simulink model "UPI_CC_3ph_4w_seq_23b"  (R2023b)
settings: Solver=FixedStepDiscrete  StartTime=0.0  StopTime=15  FixedStep=Ts_Power  MaxStep=1e-4  RelTol=1e-3
InitFcn:
  | run PI_OL_vs_UPI_CC_sec_ini;
undefined symbols (not defined in the file): C_2, DiscIntNeverNeededParam, K_i_pll, K_iv, K_p_pll, Ki_i, Kp_i, Kp_v, L_n, L_s2, L_t, L_t2, params_cc, params_pi_cc, params_pi_vc, params_vc_cc, R_d2, R_n, R_s2, R_t2, S_b, Ts_Control, Ts_Power, v_dc
libraries: spsFirstOrderFilterLib x7, spsThreePhaseSeriesRLCBranchLib x5, spsSeriesRLCLoadLib x5, spsUniversalBridgeLib x5, spsControlledVoltageSourceLib x3, spsThreePhaseVIMeasurementLib x3, eeGeneralControl x2, spsPower3phInstantaneousLib x2, spsSeriesRLCBranchLib x2, spsThreePhaseBreakerLib x2, spsRMSLib x1, simulink x1
(part 1 of 2)
settings Model: Creator=Manuel  LastModifiedBy=manba
settings SolverCC: AlgebraicLoopSolver=TrustRegion
settings DataIOCC: ReturnWorkspaceOutputs=off
settings DebuggingCC: UnconnectedInputMsg=warning  UnconnectedOutputMsg=warning  UnconnectedLineMsg=warning  ArithmeticOperatorsInVariantConditions=warning
settings ModelReferenceCC: EnableRefExpFcnMdlSchedulingChecks=on
settings SFSimCC: SimUseLocalCustomCode=off  CustomCodeUndefinedFunction=UseInterfaceOnly
settings RTWCC: RTWUseLocalCustomCode=off  DLArmComputeVersion=19.05

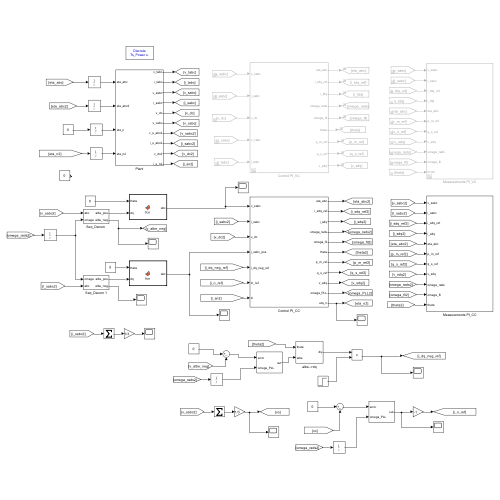
[thumbnail: Simulink's stored preview of the top-level diagram]
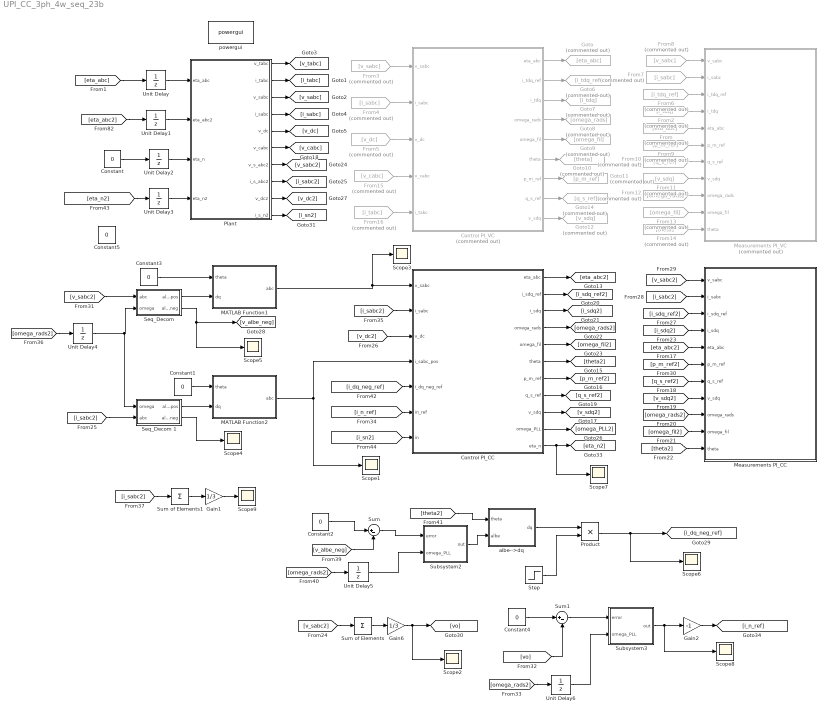
== system UPI_CC_3ph_4w_seq_23b ==
  Constant{,1..5} (6 alike) : Constant  Value=0
  Control PI_CC : Subsystem
  Control PI_VC : Subsystem  Commented=on
  From : From  Commented=on  GotoTag=eta_abc
  From10 : From  Commented=on  GotoTag=q_s_ref
  From11 : From  Commented=on  GotoTag=v_sdq
  From12 : From  Commented=on  GotoTag=omega_rads
  From13 : From  Commented=on  GotoTag=omega_fil
  From14 : From  Commented=on  GotoTag=theta
  From15 : From  Commented=on  GotoTag=v_cabc
  From16 : From  Commented=on  GotoTag=i_tabc
  From2 : From  Commented=on  GotoTag=i_tdq
  From3 : From  Commented=on  GotoTag=v_sabc
  From4 : From  Commented=on  GotoTag=i_sabc
  From5 : From  Commented=on  GotoTag=v_dc
  From6 : From  Commented=on  GotoTag=i_tdq_ref
  From7 : From  Commented=on  GotoTag=i_sabc
  From8 : From  Commented=on  GotoTag=v_sabc
  From9 : From  Commented=on  GotoTag=p_m_ref
  Gain1 : Gain  Gain=1/3
  Gain2 : Gain  Gain=-1
  Gain6 : Gain  Gain=1/3
  Goto : Goto  Commented=on  GotoTag=eta_abc
  Goto10 : Goto  Commented=on  GotoTag=theta
  Goto11 : Goto  Commented=on  GotoTag=p_m_ref
  Goto12 : Goto  Commented=on  GotoTag=v_sdq
  Goto14 : Goto  Commented=on  GotoTag=q_s_ref
  Goto6 : Goto  Commented=on  GotoTag=i_tdq_ref
  Goto7 : Goto  Commented=on  GotoTag=i_tdq
  Goto8 : Goto  Commented=on  GotoTag=omega_rads
  Goto9 : Goto  Commented=on  GotoTag=omega_fil
  MATLAB Function1 : MATLAB Function  TreatAsAtomicUnit=on
  MATLAB Function2 : MATLAB Function  TreatAsAtomicUnit=on
  Measurements PI_CC : Subsystem
  Measurements PI_VC : Subsystem  Commented=on
  Plant : Subsystem
  Product : Product
  Scope{1..9} (9 alike) : Scope
  "Seq_Decom " : Subsystem
  Seq_Decom 1 : Subsystem
  Step : Step  Time=7  SampleTime=0
  Subsystem2 : Subsystem
  Subsystem3 : Subsystem
  Sum : Sum  Inputs=|+-
  Sum of Elements : Sum  Inputs=+
  Sum of Elements1 : Sum  Inputs=+
  Sum1 : Sum  Inputs=|+-
  Unit Delay{,1..6} (7 alike) : UnitDelay  SampleTime=-1  HasFrameUpgradeWarning=on
  albe-->dq : Subsystem
  powergui : spspowerguiLib/powergui  Priority=1  SimulationMode=Discrete  SampleTime=Ts_Power  frequency=60  Iterations=50  frequencyindice=0  Pbase=100e6  ErrMax=1e-4  UnitsV=kV  UnitsW=MW  buscounter=0  FunctionMessages=off  echomessages=off  EnableUseOfTLC=off  CurrentSourceSwitches=off  DisableSnubberDevices=off  DisableRonSwitches=off  DisableVfSwitches=off  DisplayEquations=off  AutomaticDiscreteSolvers=off  SolverType=Tustin/Backward Euler (TBE)  Interpol=off  ExternalGateDelay=off  methode=off  Ts=100  x0status=blocks  SPID=on  SwTol=0  HookPort=off  NonlinearTolerance=1e-4  nMaxIteration=100  ContinueOnMaxIteration=off  RestoreLinks=warning  ResistiveCurrentMeasurement=off  Frange=[0:2:500]  Ylog=off  Xlog=on  ShowGrid=off  save=off  variable=ZData  structure=v_sabc  ZoomFFT=off  StartTime=4  cycles=5  DisplayStyle=2  fundamental=50  FreqAxis=off  MaxFrequency=10000  frequencyindicesteady=1  RmsSteady=1  display=off
  wires:
  From3/1 -> Control PI_VC/1(v_sabc)
  From4/1 -> Control PI_VC/2(i_sabc)
  From5/1 -> Control PI_VC/3(v_dc)
  Control PI_VC/1(eta_abc) -> Goto/1
  Control PI_VC/2(i_tdq_ref) -> Goto6/1
  Control PI_VC/3(i_tdq) -> Goto7/1
  Control PI_VC/4(omega_rads) -> Goto8/1
  Control PI_VC/5(omega_fil) -> Goto9/1
  Control PI_VC/6(theta) -> Goto10/1
  Control PI_VC/7(p_m_ref) -> Goto11/1
  Control PI_VC/8(q_s_ref) -> Goto14/1
  Control PI_VC/9(v_sdq) -> Goto12/1
  From/1 -> Measurements PI_VC/5(eta_abc)
  From2/1 -> Measurements PI_VC/4(i_tdq)
  From6/1 -> Measurements PI_VC/3(i_tdq_ref)
  From7/1 -> Measurements PI_VC/2(i_sabc)
  From8/1 -> Measurements PI_VC/1(v_sabc)
  From9/1 -> Measurements PI_VC/6(p_m_ref)
  From10/1 -> Measurements PI_VC/7(q_s_ref)
  From11/1 -> Measurements PI_VC/8(v_sdq)
  From12/1 -> Measurements PI_VC/9(omega_rads)
  From13/1 -> Measurements PI_VC/10(omega_fil)
  From14/1 -> Measurements PI_VC/11(theta)
  From15/1 -> Control PI_VC/4(v_cabc)
  From16/1 -> Control PI_VC/5(i_tabc)
  Plant/2(i_tabc) -> [i_tabc]
  Plant/6(v_cabc) -> [v_cabc]
  [eta_abc] -> Unit Delay/1
  Plant/7(v_s_abc2) -> [v_sabc2]
  Plant/9(v_dc2) -> [v_dc2]
  Constant/1 -> Unit Delay2/1
  Unit Delay/1 -> Plant/1(eta_abc)
  Plant/5(v_dc) -> [v_dc]
  Unit Delay1/1 -> Plant/2(eta_abc2)
  Plant/8(i_s_abc2) -> [i_sabc2]
  Plant/3(v_sabc) -> [v_sabc]
  Plant/1(v_tabc) -> [v_tabc]
  Plant/4(i_sabc) -> [i_sabc]
  Unit Delay2/1 -> Plant/3(eta_n)
  Unit Delay3/1 -> Plant/4(eta_n2)
  [eta_abc2] -> Unit Delay1/1
  Unit Delay5/1 -> Subsystem2/2(omega_PLL)
  Sum/1 -> Subsystem2/1(error)
  "Seq_Decom "/2(albe_neg) -> Scope5/1, [v_albe_neg]
  [i_dq_neg_ref] -> Control PI_CC/5(i_dq_neg_ref)
  [omega_rads2] -> Unit Delay5/1
  [v_albe_neg] -> Sum/2
  [omega_rads2] -> Measurements PI_CC/9(omega_rads)
  MATLAB Function1/1(abc) -> Control PI_CC/1(v_sabc), Scope3/1
  MATLAB Function2/1(abc) -> Scope1/1, Control PI_CC/4(i_sabc_pos)
  "Seq_Decom "/1(albe_pos) -> MATLAB Function1/2(dq)
  Control PI_CC/2(i_sdq_ref) -> [i_sdq_ref2]
  [i_sabc2] -> Seq_Decom 1/2(abc)
  Seq_Decom 1/2(albe_neg) -> Scope4/1
  [v_dc2] -> Control PI_CC/3(v_dc)
  [i_sabc2] -> Measurements PI_CC/2(i_sabc)
  Constant3/1 -> MATLAB Function1/1(theta)
  [v_sabc2] -> "Seq_Decom "/1(abc)
  [i_sabc2] -> Control PI_CC/2(i_sabc)
  [p_m_ref2] -> Measurements PI_CC/6(p_m_ref)
  [q_s_ref2] -> Measurements PI_CC/7(q_s_ref)
  [v_sdq2] -> Measurements PI_CC/8(v_sdq)
  [theta2] -> albe-->dq/1(theta)
  [i_sdq2] -> Measurements PI_CC/4(i_sdq)
  Unit Delay4/1 -> "Seq_Decom "/2(omega), Seq_Decom 1/1(omega)
  [omega_fil2] -> Measurements PI_CC/10(omega_fil)
  [eta_abc2] -> Measurements PI_CC/5(eta_abc)
  Control PI_CC/6(theta) -> [theta2]
  [omega_rads2] -> Unit Delay4/1
  Constant1/1 -> MATLAB Function2/1(theta)
  Control PI_CC/4(omega_rads) -> [omega_rads2]
  Control PI_CC/10(omega_PLL) -> [omega_PLL2]
  Control PI_CC/1(eta_abc) -> [eta_abc2]
  Seq_Decom 1/1(albe_pos) -> MATLAB Function2/2(dq)
  Control PI_CC/3(i_sdq) -> [i_sdq2]
  [theta2] -> Measurements PI_CC/11(theta)
  Control PI_CC/5(omega_fil) -> [omega_fil2]
  [i_sdq_ref2] -> Measurements PI_CC/3(i_sdq_ref)
  Control PI_CC/8(q_s_ref) -> [q_s_ref2]
  Constant2/1 -> Sum/1
  Control PI_CC/9(v_sdq) -> [v_sdq2]
  Subsystem2/1(out) -> albe-->dq/2(albe)
  [v_sabc2] -> Measurements PI_CC/1(v_sabc)
  Control PI_CC/7(p_m_ref) -> [p_m_ref2]
  Sum of Elements/1 -> Gain6/1
  Gain6/1 -> Scope2/1, [vo]
  [v_sabc2] -> Sum of Elements/1
  Constant4/1 -> Sum1/1
  [vo] -> Sum1/2
  Sum1/1 -> Subsystem3/1(error)
  [omega_rads2] -> Unit Delay6/1
  Unit Delay6/1 -> Subsystem3/2(omega_PLL)
  Subsystem3/1(out) -> Scope8/1, Gain2/1
  Plant/10(i_s_n2) -> [i_sn2]
  [i_n_ref] -> Control PI_CC/6(in_ref)
  [i_sn2] -> Control PI_CC/7(in)
  Control PI_CC/11(eta_n) -> Scope7/1, [eta_n2]
  [eta_n2] -> Unit Delay3/1
  [i_sabc2] -> Sum of Elements1/1
  Sum of Elements1/1 -> Gain1/1
  Gain1/1 -> Scope9/1
  Gain2/1 -> [i_n_ref]
  Step/1 -> Product/2
  albe-->dq/1(dq) -> Product/1
  Product/1 -> Scope6/1, [i_dq_neg_ref]

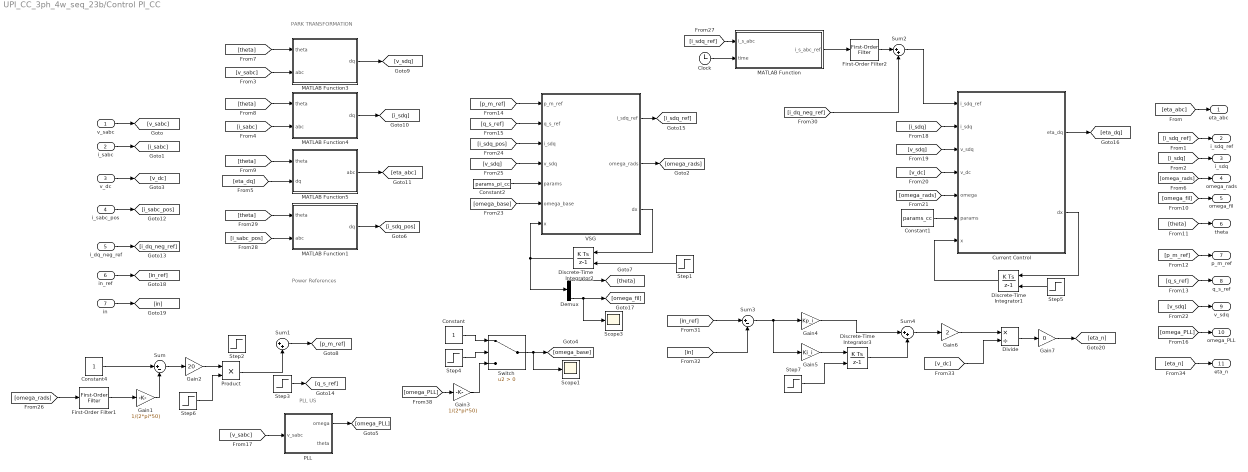
== system UPI_CC_3ph_4w_seq_23b/Control PI_CC ==
  note: PARK TRANSFORMATION
  note: Power References
  note: PLL US
  v_sabc : Inport
  i_sabc : Inport  Port=2
  v_dc : Inport  Port=3
  i_sabc_pos : Inport  Port=4
  i_dq_neg_ref : Inport  Port=5
  in_ref : Inport  Port=6
  in : Inport  Port=7
  Clock : Clock
  Constant : Constant
  Constant1 : Constant  Value=params_cc
  Constant2 : Constant  Value=params_pi_cc
  Constant4 : Constant
  Current Control : MATLAB Function  TreatAsAtomicUnit=on
  Demux : Demux
  Discrete-Time Integrator1 : DiscreteIntegrator  ExternalReset=rising  InitialCondition=[0;0]  SampleTime=Ts_Control  ICPrevOutput=DiscIntNeverNeededParam  ICPrevScaledInput=DiscIntNeverNeededParam
  Discrete-Time Integrator2 : DiscreteIntegrator  ExternalReset=rising  InitialCondition=[0;0;0;2*pi*50]  SampleTime=Ts_Control  ICPrevOutput=DiscIntNeverNeededParam  ICPrevScaledInput=DiscIntNeverNeededParam
  Discrete-Time Integrator3 : DiscreteIntegrator  ExternalReset=rising  SampleTime=Ts_Control  ICPrevOutput=DiscIntNeverNeededParam  ICPrevScaledInput=DiscIntNeverNeededParam
  Divide : Product  Inputs=*/
  First-Order Filter1 : spsFirstOrderFilterLib/First-Order Filter  FilterType=Lowpass  Tc=10e-3  Ts=Ts_Control  Initialize=on  Vac_Init=[0, 0, 60]  Vdc_Init=0  PlotResponse=off  FreqRange="[0,  200,  1]"
  First-Order Filter2 : spsFirstOrderFilterLib/First-Order Filter  FilterType=Lowpass  Tc=2.4e-3  Ts=Ts_Control  Initialize=on  Vac_Init=[0, 0, 60]  Vdc_Init=0  PlotResponse=off  FreqRange="[0,  200,  1]"
  Gain1 : Gain  Gain=1/(2*pi*50)
  Gain2 : Gain  Gain=20
  Gain3 : Gain  Gain=1/(2*pi*50)
  Gain4 : Gain  Gain=Kp_i
  Gain5 : Gain  Gain=Ki_i
  Gain6 : Gain  Gain=2
  Gain7 : Gain  Gain=0
  MATLAB Function : MATLAB Function  TreatAsAtomicUnit=on
  MATLAB Function1 : MATLAB Function  TreatAsAtomicUnit=on
  MATLAB Function3 : MATLAB Function  TreatAsAtomicUnit=on
  MATLAB Function4 : MATLAB Function  TreatAsAtomicUnit=on
  MATLAB Function5 : MATLAB Function  TreatAsAtomicUnit=on
  PLL : Subsystem
  Product : Product
  Scope1 : Scope
  Scope3 : Scope
  Step1 : Step  Time=0  SampleTime=0
  Step2 : Step  Time=4  After=0.1  SampleTime=0
  Step3 : Step  Time=12  After=0  SampleTime=0
  Step4 : Step  Time=0  SampleTime=0
  Step5 : Step  SampleTime=0
  Step6 : Step  Time=5  SampleTime=0
  Step7 : Step  SampleTime=0
  Sum : Sum  Inputs=|+-
  Sum1 : Sum  Inputs=|++
  Sum2 : Sum  Inputs=|++
  Sum3 : Sum  Inputs=|+-
  Sum4 : Sum  Inputs=|++
  Switch : Switch  Criteria=u2 > Threshold  SaturateOnIntegerOverflow=off  InputSameDT=off
  VSG : MATLAB Function  TreatAsAtomicUnit=on
  eta_abc : Outport  VectorParamsAs1DForOutWhenUnconnected=off
  i_sdq_ref : Outport  Port=2  VectorParamsAs1DForOutWhenUnconnected=off
  i_sdq : Outport  Port=3  VectorParamsAs1DForOutWhenUnconnected=off
  omega_rads : Outport  Port=4  VectorParamsAs1DForOutWhenUnconnected=off
  omega_fil : Outport  Port=5  VectorParamsAs1DForOutWhenUnconnected=off
  theta : Outport  Port=6  VectorParamsAs1DForOutWhenUnconnected=off
  p_m_ref : Outport  Port=7  VectorParamsAs1DForOutWhenUnconnected=off
  q_s_ref : Outport  Port=8  VectorParamsAs1DForOutWhenUnconnected=off
  v_sdq : Outport  Port=9  VectorParamsAs1DForOutWhenUnconnected=off
  omega_PLL : Outport  Port=10  VectorParamsAs1DForOutWhenUnconnected=off
  eta_n : Outport  Port=11  VectorParamsAs1DForOutWhenUnconnected=off
  wires:
  [theta] -> MATLAB Function4/1(theta)
  MATLAB Function5/1(abc) -> [eta_abc]
  [i_sabc] -> MATLAB Function4/2(abc)
  [eta_dq] -> MATLAB Function5/2(dq)
  MATLAB Function3/1(dq) -> [v_sdq]
  MATLAB Function4/1(dq) -> [i_sdq]
  [theta] -> MATLAB Function5/1(theta)
  [theta] -> MATLAB Function3/1(theta)
  Step3/1 -> [q_s_ref]
  [v_sabc] -> MATLAB Function3/2(abc)
  Discrete-Time Integrator2/1 -> Demux/1, VSG/7(x)
  [i_sdq_pos] -> VSG/3(i_sdq)
  Demux/4 -> Scope3/1, [omega_fil]
  Demux/1 -> [theta]
  [v_dc] -> Current Control/4(v_dc)
  [v_sdq] -> VSG/4(v_sdq)
  Constant2/1 -> VSG/5(params)
  [p_m_ref] -> VSG/1(p_m_ref)
  Constant1/1 -> Current Control/6(params)
  Current Control/1(eta_dq) -> [eta_dq]
  MATLAB Function/1(i_s_abc_ref) -> First-Order Filter2/1
  [omega_rads] -> Current Control/5(omega)
  Current Control/2(dx) -> Discrete-Time Integrator1/1
  [q_s_ref] -> VSG/2(q_s_ref)
  Discrete-Time Integrator1/1 -> Current Control/7(x)
  VSG/3(dx) -> Discrete-Time Integrator2/1
  VSG/1(i_sdq_ref) -> [i_sdq_ref]
  [v_sdq] -> Current Control/3(v_sdq)
  [i_sdq] -> Current Control/2(i_sdq)
  v_sabc/1 -> [v_sabc]
  i_sabc/1 -> [i_sabc]
  VSG/2(omega_rads) -> [omega_rads]
  v_dc/1 -> [v_dc]
  [eta_abc] -> eta_abc/1
  [i_sdq_ref] -> i_sdq_ref/1
  [i_sdq] -> i_sdq/1
  [omega_rads] -> omega_rads/1
  [omega_fil] -> omega_fil/1
  [theta] -> theta/1
  [p_m_ref] -> p_m_ref/1
  [q_s_ref] -> q_s_ref/1
  [v_sabc] -> PLL/1(v_sabc)
  [v_sdq] -> v_sdq/1
  Switch/1 -> Scope1/1, [omega_base]
  Constant/1 -> Switch/1
  Gain3/1 -> Switch/3
  [omega_PLL] -> Gain3/1
  Step4/1 -> Switch/2
  PLL/1(omega) -> [omega_PLL]
  [omega_base] -> VSG/6(omega_base)
  Step1/1 -> Discrete-Time Integrator2/2
  Step5/1 -> Discrete-Time Integrator1/2
  Gain1/1 -> Sum/2
  Constant4/1 -> Sum/1
  Sum/1 -> Gain2/1
  [omega_rads] -> First-Order Filter1/1
  Sum1/1 -> [p_m_ref]
  Gain2/1 -> Product/1
  Step6/1 -> Product/2
  Product/1 -> Sum1/2
  Clock/1 -> MATLAB Function/2(time)
  [i_sdq_ref] -> MATLAB Function/1(i_s_abc)
  First-Order Filter1/1 -> Gain1/1
  [omega_PLL] -> omega_PLL/1
  MATLAB Function1/1(dq) -> [i_sdq_pos]
  [i_sabc_pos] -> MATLAB Function1/2(abc)
  [theta] -> MATLAB Function1/1(theta)
  i_sabc_pos/1 -> [i_sabc_pos]
  i_dq_neg_ref/1 -> [i_dq_neg_ref]
  Sum2/1 -> Current Control/1(i_sdq_ref)
  First-Order Filter2/1 -> Sum2/1
  in_ref/1 -> [in_ref]
  [in_ref] -> Sum3/1
  in/1 -> [in]
  Sum3/1 -> Gain5/1, Gain4/1
  Gain5/1 -> Discrete-Time Integrator3/1
  Step7/1 -> Discrete-Time Integrator3/2
  Gain4/1 -> Sum4/1
  Discrete-Time Integrator3/1 -> Sum4/2
  Sum4/1 -> Gain6/1
  [v_dc] -> Divide/2
  Gain6/1 -> Divide/1
  Divide/1 -> Gain7/1
  [eta_n] -> eta_n/1
  [in] -> Sum3/2
  Gain7/1 -> [eta_n]
  [i_dq_neg_ref] -> Sum2/2

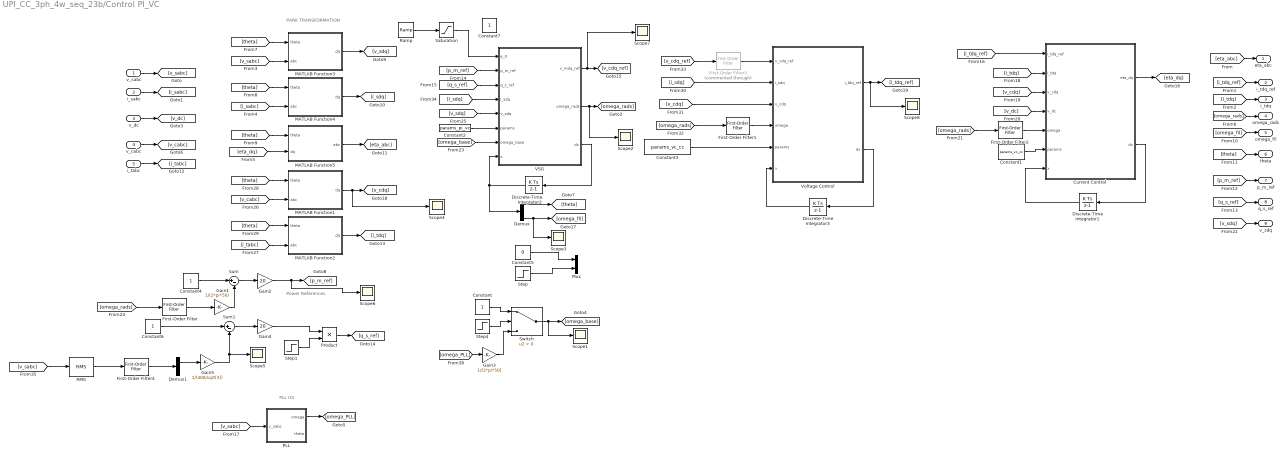
== system UPI_CC_3ph_4w_seq_23b/Control PI_VC ==
  note: PARK TRANSFORMATION
  note: Power References
  note: PLL US
  v_sabc : Inport
  i_sabc : Inport  Port=2
  v_dc : Inport  Port=3
  v_cabc : Inport  Port=4
  i_tabc : Inport  Port=5
  Constant{,4,6..7} (4 alike) : Constant
  Constant1 : Constant  Value=params_vc_cc
  Constant2 : Constant  Value=params_pi_vc
  Constant3 : Constant  Value=params_vc_cc
  Constant5 : Constant  Value=0
  Current Control : MATLAB Function  TreatAsAtomicUnit=on
  Demux : Demux
  Demux1 : Demux  Outputs=3
  Discrete-Time Integrator1 : DiscreteIntegrator  InitialCondition=[0;0]  SampleTime=Ts_Control  ICPrevOutput=DiscIntNeverNeededParam  ICPrevScaledInput=DiscIntNeverNeededParam
  Discrete-Time Integrator2 : DiscreteIntegrator  InitialCondition=[0;0;0;2*pi*50]  SampleTime=Ts_Control  ICPrevOutput=DiscIntNeverNeededParam  ICPrevScaledInput=DiscIntNeverNeededParam
  Discrete-Time Integrator3 : DiscreteIntegrator  InitialCondition=[0;0]  SampleTime=Ts_Control  ICPrevOutput=DiscIntNeverNeededParam  ICPrevScaledInput=DiscIntNeverNeededParam
  First-Order Filter{,1..2,4} (4 alike) : spsFirstOrderFilterLib/First-Order Filter  FilterType=Lowpass  Tc=10e-3  Ts=Ts_Control  Initialize=on  Vac_Init=[0, 0, 60]  Vdc_Init=0  PlotResponse=off  FreqRange="[0,  200,  1]"
  First-Order Filter3 : spsFirstOrderFilterLib/First-Order Filter  Commented=through  FilterType=Lowpass  Tc=2.4e-3  Ts=Ts_Control  Initialize=on  Vac_Init=[0, 0, 60]  Vdc_Init=0  PlotResponse=off  FreqRange="[0,  200,  1]"
  Gain1 : Gain  Gain=1/(2*pi*50)
  Gain2 : Gain  Gain=20
  Gain3 : Gain  Gain=1/(2*pi*50)
  Gain4 : Gain  Gain=20
  Gain5 : Gain  Gain=1/(400/sqrt(3))
  MATLAB Function1 : MATLAB Function  TreatAsAtomicUnit=on
  MATLAB Function2 : MATLAB Function  TreatAsAtomicUnit=on
  MATLAB Function3 : MATLAB Function  TreatAsAtomicUnit=on
  MATLAB Function4 : MATLAB Function  TreatAsAtomicUnit=on
  MATLAB Function5 : MATLAB Function  TreatAsAtomicUnit=on
  Mux : Mux  Inputs=2
  PLL : Subsystem
  Product : Product
  RMS : spsRMSLib/RMS  TrueRMS=on  Freq=50  RMSInit=230  Ts=Ts_Control
  Ramp : simulink/Sources/Ramp  slope=2  start=0  InitialOutput=0
  Saturation : Saturate  UpperLimit=1  LowerLimit=-1
  Scope{1..8} (8 alike) : Scope
  Step : Step  After=-325  SampleTime=0
  Step1 : Step  Time=0  SampleTime=0
  Step4 : Step  Time=0  SampleTime=0
  Sum : Sum  Inputs=|+-
  Sum1 : Sum  Inputs=|+-
  Switch : Switch  Criteria=u2 > Threshold  SaturateOnIntegerOverflow=off  InputSameDT=off
  VSG : MATLAB Function  TreatAsAtomicUnit=on
  Voltage Control : MATLAB Function  TreatAsAtomicUnit=on
  eta_abc : Outport  VectorParamsAs1DForOutWhenUnconnected=off
  i_tdq_ref : Outport  Port=2  VectorParamsAs1DForOutWhenUnconnected=off
  i_tdq : Outport  Port=3  VectorParamsAs1DForOutWhenUnconnected=off
  omega_rads : Outport  Port=4  VectorParamsAs1DForOutWhenUnconnected=off
  omega_fil : Outport  Port=5  VectorParamsAs1DForOutWhenUnconnected=off
  theta : Outport  Port=6  VectorParamsAs1DForOutWhenUnconnected=off
  p_m_ref : Outport  Port=7  VectorParamsAs1DForOutWhenUnconnected=off
  q_s_ref : Outport  Port=8  VectorParamsAs1DForOutWhenUnconnected=off
  v_sdq : Outport  Port=9  VectorParamsAs1DForOutWhenUnconnected=off
  wires:
  [theta] -> MATLAB Function4/1(theta)
  MATLAB Function5/1(abc) -> [eta_abc]
  [i_sabc] -> MATLAB Function4/2(abc)
  [eta_dq] -> MATLAB Function5/2(dq)
  Gain2/1 -> Scope6/1, [p_m_ref]
  MATLAB Function3/1(dq) -> [v_sdq]
  MATLAB Function4/1(dq) -> [i_sdq]
  [theta] -> MATLAB Function5/1(theta)
  [theta] -> MATLAB Function3/1(theta)
  [v_sabc] -> MATLAB Function3/2(abc)
  Discrete-Time Integrator2/1 -> Demux/1, VSG/8(x)
  Demux/4 -> Scope3/1, [omega_fil]
  Demux/1 -> [theta]
  [v_dc] -> Current Control/4(v_dc)
  Constant2/1 -> VSG/6(params)
  [p_m_ref] -> VSG/2(p_m_ref)
  Constant1/1 -> Current Control/6(params)
  Current Control/1(eta_dq) -> [eta_dq]
  [omega_rads] -> First-Order Filter2/1
  Current Control/2(dx) -> Discrete-Time Integrator1/1
  [q_s_ref] -> VSG/3(q_s_ref)
  Discrete-Time Integrator1/1 -> Current Control/7(x)
  VSG/3(dx) -> Discrete-Time Integrator2/1
  [v_cdq] -> Current Control/3(v_cdq)
  [i_tdq] -> Current Control/2(i_tdq)
  v_sabc/1 -> [v_sabc]
  i_sabc/1 -> [i_sabc]
  VSG/2(omega_rads) -> Scope2/1, [omega_rads]
  v_dc/1 -> [v_dc]
  [eta_abc] -> eta_abc/1
  [i_tdq_ref] -> i_tdq_ref/1
  [i_tdq] -> i_tdq/1
  [omega_rads] -> omega_rads/1
  [omega_fil] -> omega_fil/1
  [theta] -> theta/1
  [p_m_ref] -> p_m_ref/1
  [q_s_ref] -> q_s_ref/1
  [v_sabc] -> PLL/1(v_sabc)
  [v_sdq] -> v_sdq/1
  Switch/1 -> Scope1/1, [omega_base]
  Constant/1 -> Switch/1
  Gain3/1 -> Switch/3
  [omega_PLL] -> Gain3/1
  Step4/1 -> Switch/2
  PLL/1(omega) -> [omega_PLL]
  [omega_base] -> VSG/7(omega_base)
  i_tabc/1 -> [i_tabc]
  v_cabc/1 -> [v_cabc]
  [v_cabc] -> MATLAB Function1/2(abc)
  [theta] -> MATLAB Function1/1(theta)
  MATLAB Function2/1(dq) -> [i_tdq]
  MATLAB Function1/1(dq) -> Scope4/1, [v_cdq]
  [i_tabc] -> MATLAB Function2/2(abc)
  [theta] -> MATLAB Function2/1(theta)
  Voltage Control/2(dx) -> Discrete-Time Integrator3/1
  [i_sdq] -> Voltage Control/2(i_sdq)
  [v_cdq] -> Voltage Control/3(v_cdq)
  [omega_rads] -> First-Order Filter1/1
  Constant3/1 -> Voltage Control/5(params)
  Discrete-Time Integrator3/1 -> Voltage Control/6(x)
  Voltage Control/1(i_tdq_ref) -> Scope8/1, [i_tdq_ref]
  [v_cdq_ref] -> First-Order Filter3/1
  [i_sdq] -> VSG/4(i_sdq)
  [v_sdq] -> VSG/5(v_sdq)
  Constant5/1 -> Mux/1
  Step/1 -> Mux/2
  [omega_rads] -> First-Order Filter/1
  Gain1/1 -> Sum/2
  Sum/1 -> Gain2/1
  Sum1/1 -> Gain4/1
  VSG/1(v_mdq_ref) -> Scope7/1, [v_cdq_ref]
  [v_sabc] -> RMS/1
  RMS/1 -> First-Order Filter4/1
  Demux1/1 -> Gain5/1
  Gain5/1 -> Scope5/1, Sum1/2
  Constant4/1 -> Sum/1
  Ramp/1 -> Saturation/1
  Constant6/1 -> Sum1/1
  Product/1 -> [q_s_ref]
  Gain4/1 -> Product/1
  Step1/1 -> Product/2
  First-Order Filter/1 -> Gain1/1
  [i_tdq_ref] -> Current Control/1(i_tdq_ref)
  First-Order Filter1/1 -> Voltage Control/4(omega)
  First-Order Filter2/1 -> Current Control/5(omega)
  First-Order Filter3/1 -> Voltage Control/1(v_cdq_ref)
  First-Order Filter4/1 -> Demux1/1
  Saturation/1 -> VSG/1(e_0)

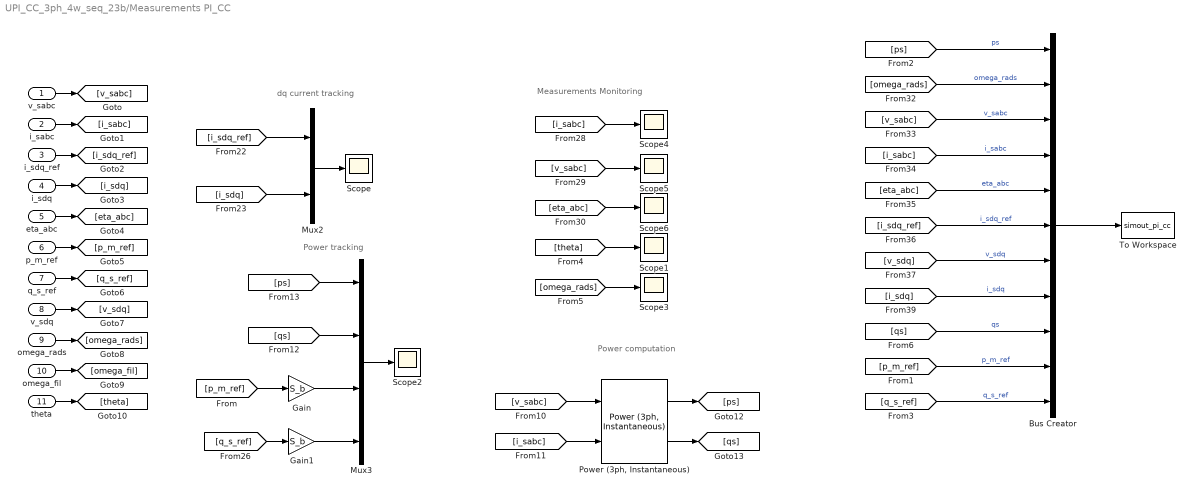
== system UPI_CC_3ph_4w_seq_23b/Measurements PI_CC ==
  note: Power computation
  note: dq current tracking
  note: Measurements Monitoring
  note: Power tracking
  v_sabc : Inport
  i_sabc : Inport  Port=2
  i_sdq_ref : Inport  Port=3
  i_sdq : Inport  Port=4
  eta_abc : Inport  Port=5
  p_m_ref : Inport  Port=6
  q_s_ref : Inport  Port=7
  v_sdq : Inport  Port=8
  omega_rads : Inport  Port=9
  omega_fil : Inport  Port=10
  theta : Inport  Port=11
  Bus Creator : BusCreator  Inputs=11
  Gain : Gain  Gain=S_b
  Gain1 : Gain  Gain=S_b
  Mux2 : Mux  Inputs=2
  Mux3 : Mux
  "Power (3ph, Instantaneous)" : spsPower3phInstantaneousLib/Power (3ph, Instantaneous)
  Scope{,1..6} (7 alike) : Scope
  To Workspace : ToWorkspace  VariableName=simout_pi_cc  SaveFormat=Timeseries  SampleTime=-1
  wires:
  [v_sdq] -> Bus Creator/7  "v_sdq"
  [i_sdq] -> Mux2/2
  [v_sabc] -> "Power (3ph, Instantaneous)"/1
  Mux2/1 -> Scope/1
  Gain1/1 -> Mux3/4
  Bus Creator/1 -> To Workspace/1
  [qs] -> Mux3/2
  [eta_abc] -> Scope6/1
  [omega_rads] -> Bus Creator/2  "omega_rads"
  [i_sdq] -> Bus Creator/8  "i_sdq"
  [i_sdq_ref] -> Mux2/1
  [p_m_ref] -> Gain/1
  [v_sabc] -> Bus Creator/3  "v_sabc"
  [ps] -> Bus Creator/1  "ps"
  [v_sabc] -> Scope5/1
  [i_sabc] -> "Power (3ph, Instantaneous)"/2
  "Power (3ph, Instantaneous)"/1 -> [ps]
  [i_sabc] -> Scope4/1
  "Power (3ph, Instantaneous)"/2 -> [qs]
  [q_s_ref] -> Gain1/1
  [eta_abc] -> Bus Creator/5  "eta_abc"
  [ps] -> Mux3/1
  [qs] -> Bus Creator/9  "qs"
  Gain/1 -> Mux3/3
  [i_sabc] -> Bus Creator/4  "i_sabc"
  Mux3/1 -> Scope2/1
  [i_sdq_ref] -> Bus Creator/6  "i_sdq_ref"
  v_sabc/1 -> [v_sabc]
  i_sabc/1 -> [i_sabc]
  i_sdq_ref/1 -> [i_sdq_ref]
  i_sdq/1 -> [i_sdq]
  eta_abc/1 -> [eta_abc]
  p_m_ref/1 -> [p_m_ref]
  q_s_ref/1 -> [q_s_ref]
  v_sdq/1 -> [v_sdq]
  omega_rads/1 -> [omega_rads]
  omega_fil/1 -> [omega_fil]
  [p_m_ref] -> Bus Creator/10  "p_m_ref"
  [q_s_ref] -> Bus Creator/11  "q_s_ref"
  theta/1 -> [theta]
  [theta] -> Scope1/1
  [omega_rads] -> Scope3/1

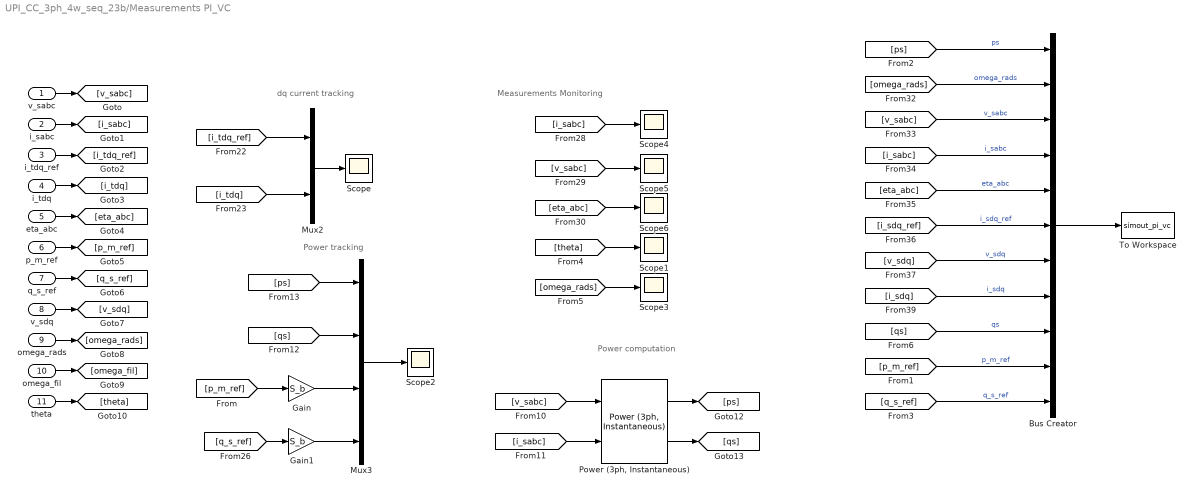
== system UPI_CC_3ph_4w_seq_23b/Measurements PI_VC ==
  note: Power computation
  note: dq current tracking
  note: Measurements Monitoring
  note: Power tracking
  v_sabc : Inport
  i_sabc : Inport  Port=2
  i_tdq_ref : Inport  Port=3
  i_tdq : Inport  Port=4
  eta_abc : Inport  Port=5
  p_m_ref : Inport  Port=6
  q_s_ref : Inport  Port=7
  v_sdq : Inport  Port=8
  omega_rads : Inport  Port=9
  omega_fil : Inport  Port=10
  theta : Inport  Port=11
  Bus Creator : BusCreator  Inputs=11
  Gain : Gain  Gain=S_b
  Gain1 : Gain  Gain=S_b
  Mux2 : Mux  Inputs=2
  Mux3 : Mux
  "Power (3ph, Instantaneous)" : spsPower3phInstantaneousLib/Power (3ph, Instantaneous)
  Scope{,1..6} (7 alike) : Scope
  To Workspace : ToWorkspace  VariableName=simout_pi_vc  SaveFormat=Timeseries  SampleTime=-1
  wires:
  [v_sdq] -> Bus Creator/7  "v_sdq"
  [i_tdq] -> Mux2/2
  [v_sabc] -> "Power (3ph, Instantaneous)"/1
  Mux2/1 -> Scope/1
  Gain1/1 -> Mux3/4
  Bus Creator/1 -> To Workspace/1
  [qs] -> Mux3/2
  [eta_abc] -> Scope6/1
  [omega_rads] -> Bus Creator/2  "omega_rads"
  [i_sdq] -> Bus Creator/8  "i_sdq"
  [i_tdq_ref] -> Mux2/1
  [p_m_ref] -> Gain/1
  [v_sabc] -> Bus Creator/3  "v_sabc"
  [ps] -> Bus Creator/1  "ps"
  [v_sabc] -> Scope5/1
  [i_sabc] -> "Power (3ph, Instantaneous)"/2
  "Power (3ph, Instantaneous)"/1 -> [ps]
  [i_sabc] -> Scope4/1
  "Power (3ph, Instantaneous)"/2 -> [qs]
  [q_s_ref] -> Gain1/1
  [eta_abc] -> Bus Creator/5  "eta_abc"
  [ps] -> Mux3/1
  [qs] -> Bus Creator/9  "qs"
  Gain/1 -> Mux3/3
  [i_sabc] -> Bus Creator/4  "i_sabc"
  Mux3/1 -> Scope2/1
  [i_sdq_ref] -> Bus Creator/6  "i_sdq_ref"
  v_sabc/1 -> [v_sabc]
  i_sabc/1 -> [i_sabc]
  i_tdq_ref/1 -> [i_tdq_ref]
  i_tdq/1 -> [i_tdq]
  eta_abc/1 -> [eta_abc]
  p_m_ref/1 -> [p_m_ref]
  q_s_ref/1 -> [q_s_ref]
  v_sdq/1 -> [v_sdq]
  omega_rads/1 -> [omega_rads]
  omega_fil/1 -> [omega_fil]
  [p_m_ref] -> Bus Creator/10  "p_m_ref"
  [q_s_ref] -> Bus Creator/11  "q_s_ref"
  theta/1 -> [theta]
  [theta] -> Scope1/1
  [omega_rads] -> Scope3/1

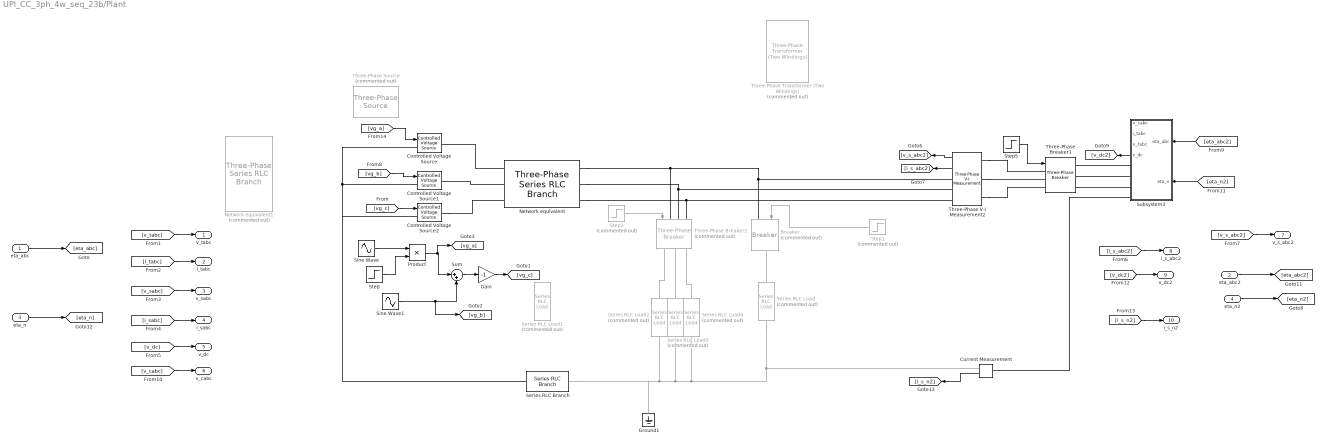
== system UPI_CC_3ph_4w_seq_23b/Plant ==
  eta_abc : Inport
  eta_abc2 : Inport  Port=2
  eta_n : Inport  Port=3
  eta_n2 : Inport  Port=4
  Breaker : spsBreakerLib/Breaker  Commented=on  InitialState=0  SwitchingTimes="[1/60  5/60]"  External=on  BreakerResistance=0.01  SnubberResistance=1e6  SnubberCapacitance=inf  Measurements=None  MoreParameters=on  NoBreakLoop=off
  Controlled Voltage Source : spsControlledVoltageSourceLib/Controlled Voltage Source  Initialize=on  Source_Type=AC  Amplitude=0  Phase=0  Frequency=0  Measurements=None
  Controlled Voltage Source1 : spsControlledVoltageSourceLib/Controlled Voltage Source  Initialize=on  Source_Type=AC  Amplitude=0  Phase=0  Frequency=0  Measurements=None
  Controlled Voltage Source2 : spsControlledVoltageSourceLib/Controlled Voltage Source  Initialize=on  Source_Type=AC  Amplitude=0  Phase=0  Frequency=0  Measurements=None
  Current Measurement : spsCurrentMeasurementLib/Current Measurement  PhasorSimulation=off  OutputType=Complex  PSBequivalent=0
  Gain : Gain  Gain=-1
  Ground1 : spsGroundLib/Ground  LConnTagsString=a
  Network equivalent : spsThreePhaseSeriesRLCBranchLib/Three-Phase Series RLC Branch  LConnTagsString=A|B|C  RConnTagsString=A|B|C  BranchType=RL  Resistance=0.34  Inductance=1e-3  Capacitance=1e-6  Measurements=None
  Network equivalent1 : spsThreePhaseSeriesRLCBranchLib/Three-Phase Series RLC Branch  Commented=on  LConnTagsString=A|B|C  RConnTagsString=A|B|C  BranchType=RL  Resistance=25  Inductance=12/(2*pi*50)  Capacitance=1e-6  Measurements=None
  Product : Product
  Series RLC Branch : spsSeriesRLCBranchLib/Series RLC Branch  LConnTagsString=__new0  RConnTagsString=__new0  BranchType=RL  Resistance=0.34  Inductance=1e-3  SetiL0=off  InitialCurrent=0  Capacitance=1e-6  Setx0=off  InitialVoltage=0  Measurements=None
  Series RLC Load : spsSeriesRLCLoadLib/Series RLC Load  Commented=on  LConnTagsString=a  RConnTagsString=__new0  NominalVoltage=230  NominalFrequency=50  ActivePower=1e3  InductivePower=1e3  CapacitivePower=0  Setx0=off  InitialVoltage=0  SetiL0=off  InitialCurrent=0  Measurements=None  LoadType=constant Z
  Series RLC Load1 : spsSeriesRLCLoadLib/Series RLC Load  Commented=on  LConnTagsString=a  RConnTagsString=__new0  NominalVoltage=230  NominalFrequency=50  ActivePower=1e3  InductivePower=1e3  CapacitivePower=0  Setx0=off  InitialVoltage=0  SetiL0=off  InitialCurrent=0  Measurements=None  LoadType=constant Z
  Series RLC Load2 : spsSeriesRLCLoadLib/Series RLC Load  Commented=on  LConnTagsString=a  RConnTagsString=__new0  NominalVoltage=230  NominalFrequency=50  ActivePower=2e3  InductivePower=500  CapacitivePower=0  Setx0=off  InitialVoltage=0  SetiL0=off  InitialCurrent=0  Measurements=None  LoadType=constant Z
  Series RLC Load3 : spsSeriesRLCLoadLib/Series RLC Load  Commented=on  LConnTagsString=a  RConnTagsString=__new0  NominalVoltage=230  NominalFrequency=50  ActivePower=2e3  InductivePower=500  CapacitivePower=0  Setx0=off  InitialVoltage=0  SetiL0=off  InitialCurrent=0  Measurements=None  LoadType=constant Z
  Series RLC Load4 : spsSeriesRLCLoadLib/Series RLC Load  Commented=on  LConnTagsString=a  RConnTagsString=__new0  NominalVoltage=230  NominalFrequency=50  ActivePower=2e3  InductivePower=500  CapacitivePower=0  Setx0=off  InitialVoltage=0  SetiL0=off  InitialCurrent=0  Measurements=None  LoadType=constant Z
  Sine Wave : Sin  Amplitude=230*sqrt(2)  Frequency=2*pi*50  SampleTime=Ts_Control
  Sine Wave1 : Sin  Amplitude=230*sqrt(2)  Frequency=2*pi*50  Phase=-2*pi/3  SampleTime=Ts_Control
  Step : Step  Time=5  Before=1  After=0.9  SampleTime=0
  Step1 : Step  Commented=on  Time=10  SampleTime=0
  Step2 : Step  Commented=on  Time=3  SampleTime=0
  Step5 : Step  SampleTime=0
  Subsystem3 : Subsystem
  Sum : Sum  Inputs=|++
  Three-Phase Transformer (Two Windings) : spsThreePhaseTransformerTwoWindingsLib/Three-Phase Transformer (Two Windings)  Commented=on  Winding1Connection=Yn  Winding2Connection=Yn  CoreType=Three single-phase transformers  SetSaturation=off  Hysteresis=off  DataFile='hysteresis'  SetInitialFlux=off  Measurements=None  UNITS=pu  NominalPower=[ 125e3 , 50 ]  Winding1=[ 400 , 0.002 , 0.08 ]  Winding2=[ 400 , 0.002 , 0.08 ]  Rm=500  Lm=500  L0=0.5  Saturation=[ 0,0 ; 0.0024,1.2 ; 1.0,1.52 ]  InitialFluxes=[ 0.8 , -0.8 , 0.7 ]  BreakLoop=off  DiscreteSolver=Trapezoidal iterative  DataType=off  TransfoNumber=1
  Three-Phase V-I Measurement2 : spsThreePhaseVIMeasurementLib/Three-Phase V-I Measurement  VoltageMeasurement=phase-to-ground  SetLabelV=off  LabelV=Vabc  Vpu=off  VpuLL=off  CurrentMeasurement=yes  SetLabelI=off  LabelI=Iabc  Ipu=off  Pbase=100e6  Vbase=500e3  OutputType=Complex  PhasorSimulation=off  PSBequivalent=0
  Three-Phase Breaker1 : spsThreePhaseBreakerLib/Three-Phase Breaker  InitialState=open  SwitchA=on  SwitchB=on  SwitchC=on  SwitchTimes="[1/60  5/60]"  External=on  BreakerResistance=0.01  SnubberResistance=1e6  SnubberCapacitance=inf  Measurements=None
  Three-Phase Breaker2 : spsThreePhaseBreakerLib/Three-Phase Breaker  Commented=on  InitialState=open  SwitchA=on  SwitchB=on  SwitchC=on  SwitchTimes="[1/60  5/60]"  External=on  BreakerResistance=0.01  SnubberResistance=1e6  SnubberCapacitance=inf  Measurements=None
  Three-Phase Source : spsThreePhaseSourceLib/Three-Phase Source  Commented=on  InternalConnection=Yn  VoltagePhases=off  Voltage=400  PhaseAngle=0  Voltage_phases=[25e3 25e3 25e3]/sqrt(3)  PhaseAngles_phases=[0 -120 +120]  Frequency=50  NonIdealSource=on  SpecifyImpedance=off  Resistance=0.8929  Inductance=16.58e-3  ShortCircuitLevel=100e6  BaseVoltage=25e3  XRratio=7  BusType=swing  Pref=10e3  Qref=0  Prefabc=[10e3, 10e3, 10e3]  Qrefabc=[0, 0, 0]  Qmin=-inf  Qmax=inf
  v_tabc : Outport  VectorParamsAs1DForOutWhenUnconnected=off
  i_tabc : Outport  Port=2  VectorParamsAs1DForOutWhenUnconnected=off
  v_sabc : Outport  Port=3  VectorParamsAs1DForOutWhenUnconnected=off
  i_sabc : Outport  Port=4  VectorParamsAs1DForOutWhenUnconnected=off
  v_dc : Outport  Port=5  VectorParamsAs1DForOutWhenUnconnected=off
  v_cabc : Outport  Port=6  VectorParamsAs1DForOutWhenUnconnected=off
  v_s_abc2 : Outport  Port=7  VectorParamsAs1DForOutWhenUnconnected=off
  i_s_abc2 : Outport  Port=8  VectorParamsAs1DForOutWhenUnconnected=off
  v_dc2 : Outport  Port=9  VectorParamsAs1DForOutWhenUnconnected=off
  i_s_n2 : Outport  Port=10  VectorParamsAs1DForOutWhenUnconnected=off
  wires:
  [v_tabc] -> v_tabc/1
  [i_tabc] -> i_tabc/1
  [v_sabc] -> v_sabc/1
  [i_sabc] -> i_sabc/1
  eta_abc/1 -> [eta_abc]
  [v_dc] -> v_dc/1
  [v_cabc] -> v_cabc/1
  Three-Phase V-I Measurement2/2 -> [i_s_abc2]
  Three-Phase V-I Measurement2/1 -> [v_s_abc2]
  Step5/1 -> Three-Phase Breaker1/1
  [i_s_abc2] -> i_s_abc2/1
  [v_s_abc2] -> v_s_abc2/1
  eta_abc2/1 -> [eta_abc2]
  eta_n/1 -> [eta_n]
  [v_dc2] -> v_dc2/1
  [eta_abc2] -> Subsystem3/1(eta_abc)
  Subsystem3/4(v_dc) -> [v_dc2]
  eta_n2/1 -> [eta_n2]
  [eta_n2] -> Subsystem3/2(eta_n)
  Step1/1 -> Breaker/1
  Step2/1 -> Three-Phase Breaker2/1
  Current Measurement/1 -> [i_s_n2]
  [i_s_n2] -> i_s_n2/1
  Sine Wave1/1 -> [vg_b], Sum/2
  Sum/1 -> Gain/1
  [vg_c] -> Controlled Voltage Source2/1
  [vg_b] -> Controlled Voltage Source1/1
  Sine Wave/1 -> Product/1
  Product/1 -> [vg_a], Sum/1
  Step/1 -> Product/2
  [vg_a] -> Controlled Voltage Source/1
  Gain/1 -> [vg_c]
  connections:
  Series RLC Load/RConn1 -- Series RLC Load4/RConn1 -- Series RLC Load3/RConn1 -- Series RLC Load2/RConn1 -- Series RLC Branch/RConn1 -- Ground1/LConn1 -- Current Measurement/RConn1
  Subsystem3/RConn2 -- Three-Phase Breaker1/RConn2
  Subsystem3/RConn3 -- Three-Phase Breaker1/RConn3
  Subsystem3/RConn1 -- Three-Phase Breaker1/RConn1
  Three-Phase V-I Measurement2/LConn2 -- Three-Phase Breaker1/LConn2
  Three-Phase V-I Measurement2/LConn3 -- Three-Phase Breaker1/LConn3
  Three-Phase V-I Measurement2/LConn1 -- Three-Phase Breaker1/LConn1
  Network equivalent/RConn2 -- Three-Phase V-I Measurement2/RConn2 -- Three-Phase Breaker2/LConn2
  Network equivalent/RConn3 -- Three-Phase V-I Measurement2/RConn3 -- Three-Phase Breaker2/LConn3
  Network equivalent/RConn1 -- Three-Phase Breaker2/LConn1 -- Three-Phase V-I Measurement2/RConn1 -- Breaker/LConn1
  Series RLC Load/LConn1 -- Breaker/RConn1
  Series RLC Load3/LConn1 -- Three-Phase Breaker2/RConn2
  Series RLC Load2/LConn1 -- Three-Phase Breaker2/RConn1
  Series RLC Load4/LConn1 -- Three-Phase Breaker2/RConn3
  Subsystem3/RConn4 -- Current Measurement/LConn1
  Controlled Voltage Source/LConn1 -- Controlled Voltage Source1/LConn1 -- Controlled Voltage Source2/LConn1 -- Series RLC Branch/LConn1
  Network equivalent/LConn2 -- Controlled Voltage Source1/RConn1
  Controlled Voltage Source2/RConn1 -- Network equivalent/LConn3
  Network equivalent/LConn1 -- Controlled Voltage Source/RConn1

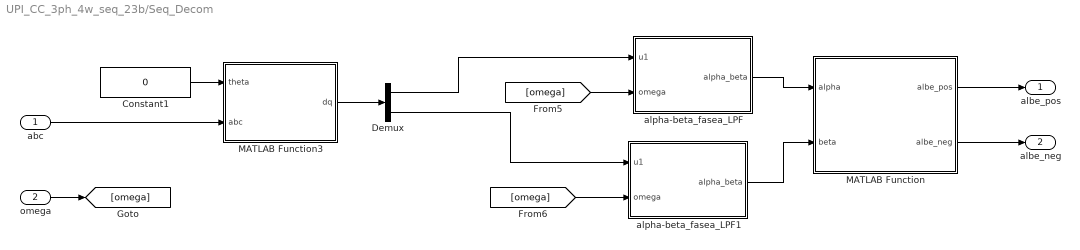
== system UPI_CC_3ph_4w_seq_23b/Seq_Decom  ==
  abc : Inport
  omega : Inport  Port=2
  Constant1 : Constant  Value=0  SampleTime=50e-6
  Demux : Demux  Outputs=2
  MATLAB Function : MATLAB Function  TreatAsAtomicUnit=on
  MATLAB Function3 : MATLAB Function  TreatAsAtomicUnit=on
  alpha-beta_fasea_LPF : Subsystem
  alpha-beta_fasea_LPF1 : Subsystem
  albe_pos : Outport
  albe_neg : Outport  Port=2
  wires:
  [omega] -> alpha-beta_fasea_LPF1/2(omega)
  MATLAB Function3/1(dq) -> Demux/1
  Demux/1 -> alpha-beta_fasea_LPF/1(u1)
  alpha-beta_fasea_LPF1/1(alpha_beta) -> MATLAB Function/2(beta)
  alpha-beta_fasea_LPF/1(alpha_beta) -> MATLAB Function/1(alpha)
  Demux/2 -> alpha-beta_fasea_LPF1/1(u1)
  abc/1 -> MATLAB Function3/2(abc)
  Constant1/1 -> MATLAB Function3/1(theta)
  [omega] -> alpha-beta_fasea_LPF/2(omega)
  MATLAB Function/2(albe_neg) -> albe_neg/1
  MATLAB Function/1(albe_pos) -> albe_pos/1
  omega/1 -> [omega]

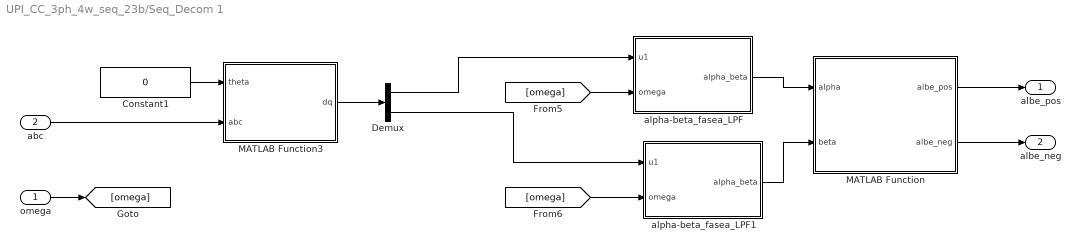
== system UPI_CC_3ph_4w_seq_23b/Seq_Decom 1 ==
  omega : Inport
  abc : Inport  Port=2
  Constant1 : Constant  Value=0  SampleTime=50e-6
  Demux : Demux  Outputs=2
  MATLAB Function : MATLAB Function  TreatAsAtomicUnit=on
  MATLAB Function3 : MATLAB Function  TreatAsAtomicUnit=on
  alpha-beta_fasea_LPF : Subsystem
  alpha-beta_fasea_LPF1 : Subsystem
  albe_pos : Outport
  albe_neg : Outport  Port=2
  wires:
  omega/1 -> [omega]
  MATLAB Function/1(albe_pos) -> albe_pos/1
  MATLAB Function/2(albe_neg) -> albe_neg/1
  [omega] -> alpha-beta_fasea_LPF/2(omega)
  Constant1/1 -> MATLAB Function3/1(theta)
  abc/1 -> MATLAB Function3/2(abc)
  Demux/2 -> alpha-beta_fasea_LPF1/1(u1)
  alpha-beta_fasea_LPF/1(alpha_beta) -> MATLAB Function/1(alpha)
  alpha-beta_fasea_LPF1/1(alpha_beta) -> MATLAB Function/2(beta)
  Demux/1 -> alpha-beta_fasea_LPF/1(u1)
  MATLAB Function3/1(dq) -> Demux/1
  [omega] -> alpha-beta_fasea_LPF1/2(omega)

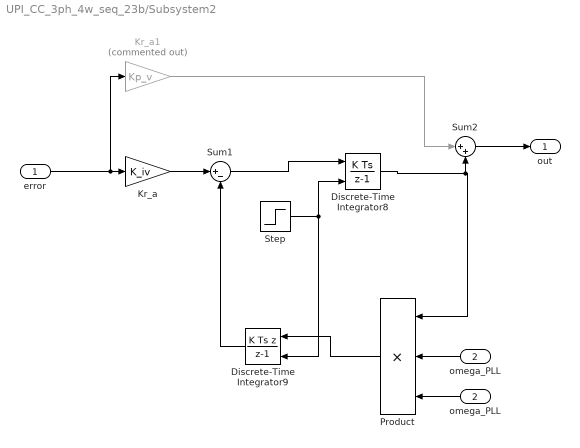
== system UPI_CC_3ph_4w_seq_23b/Subsystem2 ==
  error : Inport
  omega_PLL : Inport  Port=2
  Discrete-Time Integrator8 : DiscreteIntegrator  ExternalReset=rising  InitialCondition=[0,0]  SampleTime=-1  ICPrevOutput=DiscIntNeverNeededParam  ICPrevScaledInput=DiscIntNeverNeededParam
  Discrete-Time Integrator9 : DiscreteIntegrator  IntegratorMethod=Integration: Backward Euler  ExternalReset=rising  InitialCondition=[0,0]  SampleTime=-1  ICPrevOutput=DiscIntNeverNeededParam  ICPrevScaledInput=DiscIntNeverNeededParam
  Kr_a : Gain  Gain=K_iv
  Kr_a1 : Gain  Commented=on  Gain=Kp_v
  Product : Product  Inputs=3
  Step : Step  Time=7  SampleTime=0
  Sum1 : Sum  Inputs=|+-
  Sum2 : Sum  Inputs=|++
  "omega_PLL " : InportShadow  Port=2
  out : Outport  VectorParamsAs1DForOutWhenUnconnected=off
  wires:
  Sum2/1 -> out/1
  Kr_a1/1 -> Sum2/1
  Discrete-Time Integrator9/1 -> Sum1/2
  error/1 -> Kr_a/1, Kr_a1/1
  Product/1 -> Discrete-Time Integrator9/1
  Discrete-Time Integrator8/1 -> Product/1, Sum2/2
  Sum1/1 -> Discrete-Time Integrator8/1
  Kr_a/1 -> Sum1/1
  omega_PLL/1 -> Product/2
  "omega_PLL "/1 -> Product/3
  Step/1 -> Discrete-Time Integrator8/2, Discrete-Time Integrator9/2

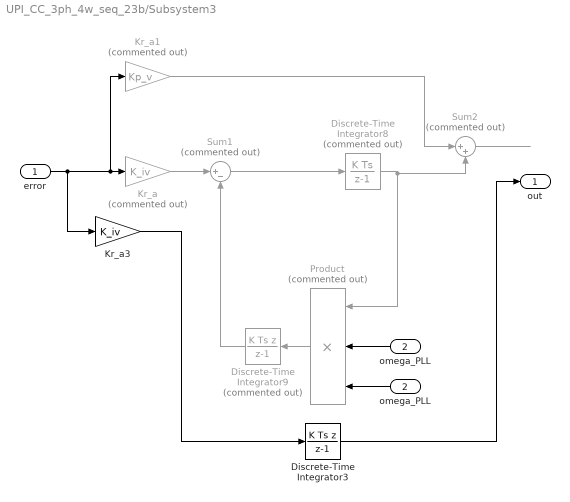
== system UPI_CC_3ph_4w_seq_23b/Subsystem3 ==
  error : Inport
  omega_PLL : Inport  Port=2
  Discrete-Time Integrator3 : DiscreteIntegrator  IntegratorMethod=Integration: Backward Euler  SampleTime=Ts_Control  ICPrevOutput=DiscIntNeverNeededParam  ICPrevScaledInput=DiscIntNeverNeededParam
  Discrete-Time Integrator8 : DiscreteIntegrator  Commented=on  InitialCondition=[0,0]  SampleTime=-1  ICPrevOutput=DiscIntNeverNeededParam  ICPrevScaledInput=DiscIntNeverNeededParam
  Discrete-Time Integrator9 : DiscreteIntegrator  Commented=on  IntegratorMethod=Integration: Backward Euler  InitialCondition=[0,0]  SampleTime=-1  ICPrevOutput=DiscIntNeverNeededParam  ICPrevScaledInput=DiscIntNeverNeededParam
  Kr_a : Gain  Commented=on  Gain=K_iv
  Kr_a1 : Gain  Commented=on  Gain=Kp_v
  Kr_a3 : Gain  Gain=K_iv
  Product : Product  Commented=on  Inputs=3
  Sum1 : Sum  Commented=on  Inputs=|+-
  Sum2 : Sum  Commented=on  Inputs=|++
  "omega_PLL " : InportShadow  Port=2
  out : Outport  VectorParamsAs1DForOutWhenUnconnected=off
  wires:
  Discrete-Time Integrator3/1 -> out/1
  Kr_a3/1 -> Discrete-Time Integrator3/1
  Sum2/1 -> ?
  Kr_a1/1 -> Sum2/1
  Discrete-Time Integrator9/1 -> Sum1/2
  error/1 -> Kr_a/1, Kr_a1/1, Kr_a3/1
  Product/1 -> Discrete-Time Integrator9/1
  Discrete-Time Integrator8/1 -> Product/1, Sum2/2
  Sum1/1 -> Discrete-Time Integrator8/1
  Kr_a/1 -> Sum1/1
  omega_PLL/1 -> Product/2
  "omega_PLL "/1 -> Product/3

== system UPI_CC_3ph_4w_seq_23b/albe-->dq ==
  theta : Inport
  albe : Inport  Port=2
  Constant : Constant  Value=0
  MATLAB Function1 : MATLAB Function  TreatAsAtomicUnit=on
  MATLAB Function5 : MATLAB Function  TreatAsAtomicUnit=on
  dq : Outport
  wires:
  Constant/1 -> MATLAB Function5/1(theta)
  MATLAB Function5/1(abc) -> MATLAB Function1/2(abc)
  theta/1 -> MATLAB Function1/1(theta)
  albe/1 -> MATLAB Function5/2(dq)
  MATLAB Function1/1(dq) -> dq/1

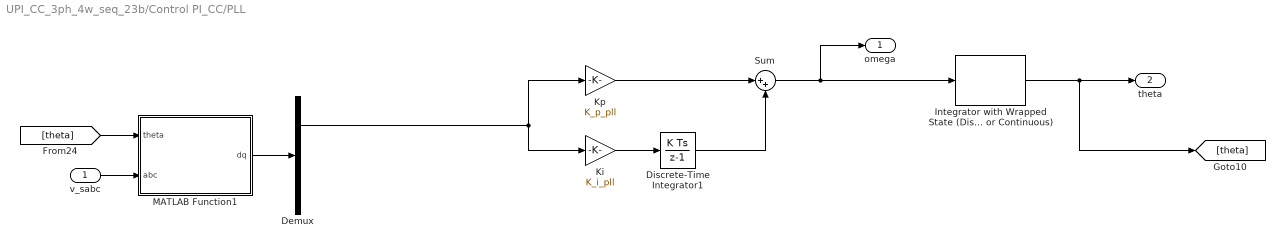
== system UPI_CC_3ph_4w_seq_23b/Control PI_CC/PLL ==
  v_sabc : Inport
  Demux : Demux  Outputs=2
  Discrete-Time Integrator1 : DiscreteIntegrator  SampleTime=Ts_Control  ICPrevOutput=DiscIntNeverNeededParam  ICPrevScaledInput=DiscIntNeverNeededParam
  Integrator with Wrapped State (Discrete or Continuous) : eeGeneralControl/Integrator with Wrapped State (Discrete or Continuous)  LabelModeActiveChoice=Discrete  WrappedStateUpperValue=2*pi  WrappedStateLowerValue=0  x0=0  Ts=Ts_Control
  Ki : Gain  Gain=K_i_pll
  Kp : Gain  Gain=K_p_pll
  MATLAB Function1 : MATLAB Function  TreatAsAtomicUnit=on
  Sum : Sum  Inputs=|++
  omega : Outport  VectorParamsAs1DForOutWhenUnconnected=off
  theta : Outport  Port=2  VectorParamsAs1DForOutWhenUnconnected=off
  wires:
  MATLAB Function1/1(dq) -> Demux/1
  v_sabc/1 -> MATLAB Function1/2(abc)
  [theta] -> MATLAB Function1/1(theta)
  Ki/1 -> Discrete-Time Integrator1/1
  Kp/1 -> Sum/1
  Discrete-Time Integrator1/1 -> Sum/2
  Sum/1 -> Integrator with Wrapped State (Discrete or Continuous)/1, omega/1
  Integrator with Wrapped State (Discrete or Continuous)/1 -> [theta], theta/1
  Demux/1 -> Ki/1, Kp/1

== system UPI_CC_3ph_4w_seq_23b/Control PI_VC/PLL ==
  v_sabc : Inport
  Demux : Demux  Outputs=2
  Discrete-Time Integrator1 : DiscreteIntegrator  SampleTime=Ts_Control  ICPrevOutput=DiscIntNeverNeededParam  ICPrevScaledInput=DiscIntNeverNeededParam
  Integrator with Wrapped State (Discrete or Continuous) : eeGeneralControl/Integrator with Wrapped State (Discrete or Continuous)  LabelModeActiveChoice=Discrete  WrappedStateUpperValue=2*pi  WrappedStateLowerValue=0  x0=0  Ts=Ts_Control
  Ki : Gain  Gain=K_i_pll
  Kp : Gain  Gain=K_p_pll
  MATLAB Function1 : MATLAB Function  TreatAsAtomicUnit=on
  Sum : Sum  Inputs=|++
  omega : Outport  VectorParamsAs1DForOutWhenUnconnected=off
  theta : Outport  Port=2  VectorParamsAs1DForOutWhenUnconnected=off
  wires:
  MATLAB Function1/1(dq) -> Demux/1
  v_sabc/1 -> MATLAB Function1/2(abc)
  [theta] -> MATLAB Function1/1(theta)
  Ki/1 -> Discrete-Time Integrator1/1
  Kp/1 -> Sum/1
  Discrete-Time Integrator1/1 -> Sum/2
  Sum/1 -> Integrator with Wrapped State (Discrete or Continuous)/1, omega/1
  Integrator with Wrapped State (Discrete or Continuous)/1 -> [theta], theta/1
  Demux/1 -> Ki/1, Kp/1

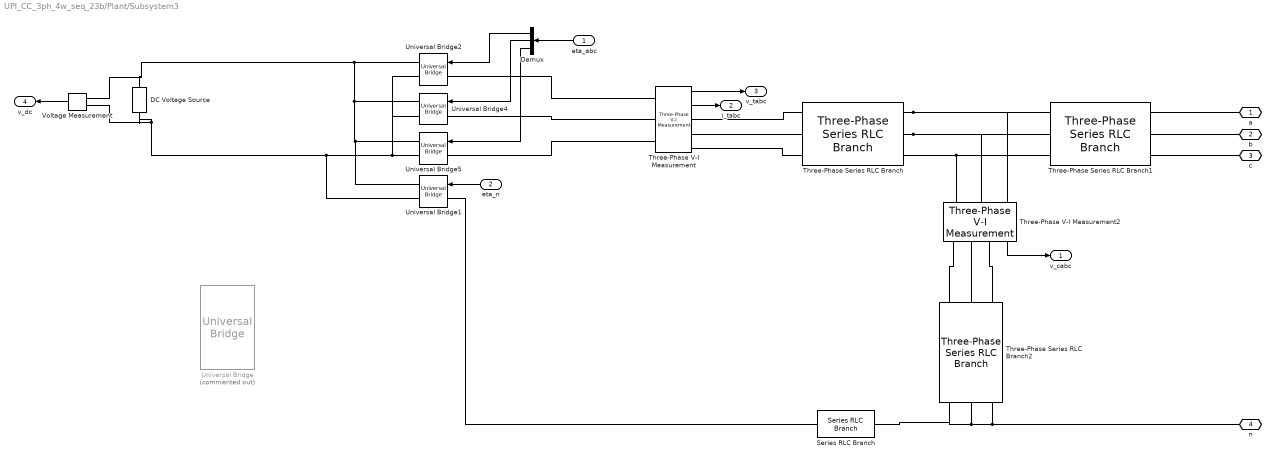
== system UPI_CC_3ph_4w_seq_23b/Plant/Subsystem3 ==
  eta_abc : Inport
  eta_n : Inport  Port=2
  DC Voltage Source : spsDCVoltageSourceLib/DC Voltage Source  Amplitude=v_dc  Measurements=None
  Demux : Demux  Outputs=3
  Series RLC Branch : spsSeriesRLCBranchLib/Series RLC Branch  LConnTagsString=__new0  RConnTagsString=__new0  BranchType=RL  Resistance=R_n  Inductance=L_n  SetiL0=off  InitialCurrent=0  Capacitance=1e-6  Setx0=off  InitialVoltage=0  Measurements=None
  Three-Phase Series RLC Branch : spsThreePhaseSeriesRLCBranchLib/Three-Phase Series RLC Branch  LConnTagsString=A|B|C  RConnTagsString=A|B|C  BranchType=RL  Resistance=R_t2  Inductance=L_t2  Capacitance=1e-6  Measurements=None
  Three-Phase Series RLC Branch1 : spsThreePhaseSeriesRLCBranchLib/Three-Phase Series RLC Branch  LConnTagsString=A|B|C  RConnTagsString=A|B|C  BranchType=RL  Resistance=R_s2  Inductance=L_s2  Capacitance=1e-6  Measurements=None
  Three-Phase Series RLC Branch2 : spsThreePhaseSeriesRLCBranchLib/Three-Phase Series RLC Branch  LConnTagsString=A|B|C  RConnTagsString=A|B|C  BranchType=RC  Resistance=R_d2  Inductance=L_t  Capacitance=C_2  Measurements=None
  Three-Phase V-I Measurement : spsThreePhaseVIMeasurementLib/Three-Phase V-I Measurement  VoltageMeasurement=phase-to-ground  SetLabelV=off  LabelV=Vabc  Vpu=off  VpuLL=off  CurrentMeasurement=yes  SetLabelI=off  LabelI=Iabc  Ipu=off  Pbase=100e6  Vbase=500e3  OutputType=Complex  PhasorSimulation=off  PSBequivalent=0
  Three-Phase V-I Measurement2 : spsThreePhaseVIMeasurementLib/Three-Phase V-I Measurement  VoltageMeasurement=phase-to-ground  SetLabelV=off  LabelV=Vabc  Vpu=off  VpuLL=off  CurrentMeasurement=no  SetLabelI=off  LabelI=Iabc  Ipu=off  Pbase=100e6  Vbase=500e3  OutputType=Complex  PhasorSimulation=off  PSBequivalent=0
  Universal Bridge : spsUniversalBridgeLib/Universal Bridge  Commented=on  Arms=3  SnubberResistance=1e5  SnubberCapacitance=inf  Device=Average-model based VSC  Ron=1e-3  Lon=0  ForwardVoltages="[  0  0  ]"  ForwardVoltage=0  GTOparameters=[ 10e-6 , 20e-6 ]  IGBTparameters=[ 1e-6 , 2e-6 ]  Measurements=None  Measurements_2=None  converterType=Rectifier
  Universal Bridge{1..2,4..5} (4 alike) : spsUniversalBridgeLib/Universal Bridge  Arms=1  SnubberResistance=1e5  SnubberCapacitance=inf  Device=Average-model based VSC  Ron=1e-3  Lon=0  ForwardVoltages="[  0  0  ]"  ForwardVoltage=0  GTOparameters=[ 10e-6 , 20e-6 ]  IGBTparameters=[ 1e-6 , 2e-6 ]  Measurements=None  Measurements_2=None  converterType=Rectifier
  Voltage Measurement : spsVoltageMeasurementLib/Voltage Measurement  PhasorSimulation=off  OutputType=Complex  PSBequivalent=0
  a : PMIOPort  Side=Right
  b : PMIOPort  Port=2  Side=Right
  c : PMIOPort  Port=3  Side=Right
  n : PMIOPort  Port=4  Side=Right
  v_cabc : Outport
  i_tabc : Outport  Port=2
  v_tabc : Outport  Port=3
  v_dc : Outport  Port=4
  wires:
  eta_n/1 -> Universal Bridge1/1
  Demux/3 -> Universal Bridge5/1
  Demux/2 -> Universal Bridge4/1
  Demux/1 -> Universal Bridge2/1
  Voltage Measurement/1 -> v_dc/1
  eta_abc/1 -> Demux/1
  Three-Phase V-I Measurement/1 -> v_tabc/1
  Three-Phase V-I Measurement2/1 -> v_cabc/1
  Three-Phase V-I Measurement/2 -> i_tabc/1
  connections:
  Universal Bridge1/LConn1 -- Series RLC Branch/LConn1
  Three-Phase Series RLC Branch1/RConn3 -- c/RConn1
  b/RConn1 -- Three-Phase Series RLC Branch1/RConn2
  a/RConn1 -- Three-Phase Series RLC Branch1/RConn1
  Three-Phase V-I Measurement/LConn3 -- Universal Bridge5/LConn1
  n/RConn1 -- Three-Phase Series RLC Branch2/RConn2 -- Three-Phase Series RLC Branch2/RConn1 -- Series RLC Branch/RConn1 -- Three-Phase Series RLC Branch2/RConn3
  Three-Phase V-I Measurement2/RConn1 -- Three-Phase Series RLC Branch2/LConn3
  Three-Phase Series RLC Branch/RConn1 -- Three-Phase V-I Measurement2/LConn1 -- Three-Phase Series RLC Branch1/LConn1
  Three-Phase V-I Measurement/LConn1 -- Universal Bridge2/LConn1
  Three-Phase Series RLC Branch/LConn2 -- Three-Phase V-I Measurement/RConn2
  Three-Phase Series RLC Branch/RConn2 -- Three-Phase V-I Measurement2/LConn2 -- Three-Phase Series RLC Branch1/LConn2
  Three-Phase Series RLC Branch2/LConn1 -- Three-Phase V-I Measurement2/RConn3
  Three-Phase Series RLC Branch2/LConn2 -- Three-Phase V-I Measurement2/RConn2
  Universal Bridge1/RConn2 -- Universal Bridge5/RConn2 -- Universal Bridge4/RConn2 -- Universal Bridge2/RConn2 -- Voltage Measurement/LConn2 -- DC Voltage Source/LConn1
  Universal Bridge1/RConn1 -- Universal Bridge5/RConn1 -- Universal Bridge4/RConn1 -- Voltage Measurement/LConn1 -- DC Voltage Source/RConn1 -- Universal Bridge2/RConn1
  Three-Phase Series RLC Branch1/LConn3 -- Three-Phase Series RLC Branch/RConn3 -- Three-Phase V-I Measurement2/LConn3
  Three-Phase V-I Measurement/RConn1 -- Three-Phase Series RLC Branch/LConn1
  Three-Phase V-I Measurement/LConn2 -- Universal Bridge4/LConn1
  Three-Phase V-I Measurement/RConn3 -- Three-Phase Series RLC Branch/LConn3

== system UPI_CC_3ph_4w_seq_23b/Seq_Decom /alpha-beta_fasea_LPF ==
  u1 : Inport
  omega : Inport  Port=2
  Gain2 : Gain  Gain=2
  MATLAB Function2 : MATLAB Function  TreatAsAtomicUnit=on
  Mux1 : Mux  Inputs=2
  Unit Delay3 : UnitDelay  SampleTime=50e-6  HasFrameUpgradeWarning=on
  Unit Delay4 : UnitDelay  SampleTime=50e-6  HasFrameUpgradeWarning=on
  Unit Delay5 : UnitDelay  SampleTime=50e-6  HasFrameUpgradeWarning=on
  "u1  " : InportShadow
  alpha_beta : Outport
  wires:
  Unit Delay3/1 -> MATLAB Function2/4(y1_k_1)
  MATLAB Function2/1(y1_k) -> Unit Delay3/1
  Unit Delay5/1 -> MATLAB Function2/2(u1_k_1)
  Unit Delay4/1 -> MATLAB Function2/5(y2_k_1)
  MATLAB Function2/2(y2_k) -> Gain2/1, Unit Delay4/1
  "u1  "/1 -> Unit Delay5/1
  omega/1 -> MATLAB Function2/3(omega)
  Gain2/1 -> Mux1/2
  u1/1 -> Mux1/1, MATLAB Function2/1(u1)
  Mux1/1 -> alpha_beta/1

== system UPI_CC_3ph_4w_seq_23b/Seq_Decom /alpha-beta_fasea_LPF1 ==
  u1 : Inport
  omega : Inport  Port=2
  Gain2 : Gain  Gain=2
  MATLAB Function2 : MATLAB Function  TreatAsAtomicUnit=on
  Mux1 : Mux  Inputs=2
  Unit Delay3 : UnitDelay  SampleTime=50e-6  HasFrameUpgradeWarning=on
  Unit Delay4 : UnitDelay  SampleTime=50e-6  HasFrameUpgradeWarning=on
  Unit Delay5 : UnitDelay  SampleTime=50e-6  HasFrameUpgradeWarning=on
  "u1  " : InportShadow
  alpha_beta : Outport
  wires:
  Mux1/1 -> alpha_beta/1
  u1/1 -> MATLAB Function2/1(u1), Mux1/1
  Gain2/1 -> Mux1/2
  omega/1 -> MATLAB Function2/3(omega)
  "u1  "/1 -> Unit Delay5/1
  MATLAB Function2/2(y2_k) -> Unit Delay4/1, Gain2/1
  Unit Delay4/1 -> MATLAB Function2/5(y2_k_1)
  Unit Delay5/1 -> MATLAB Function2/2(u1_k_1)
  MATLAB Function2/1(y1_k) -> Unit Delay3/1
  Unit Delay3/1 -> MATLAB Function2/4(y1_k_1)

== system UPI_CC_3ph_4w_seq_23b/Seq_Decom 1/alpha-beta_fasea_LPF ==
  u1 : Inport
  omega : Inport  Port=2
  Gain2 : Gain  Gain=2
  MATLAB Function2 : MATLAB Function  TreatAsAtomicUnit=on
  Mux1 : Mux  Inputs=2
  Unit Delay3 : UnitDelay  SampleTime=50e-6  HasFrameUpgradeWarning=on
  Unit Delay4 : UnitDelay  SampleTime=50e-6  HasFrameUpgradeWarning=on
  Unit Delay5 : UnitDelay  SampleTime=50e-6  HasFrameUpgradeWarning=on
  "u1  " : InportShadow
  alpha_beta : Outport
  wires:
  Mux1/1 -> alpha_beta/1
  u1/1 -> MATLAB Function2/1(u1), Mux1/1
  Gain2/1 -> Mux1/2
  omega/1 -> MATLAB Function2/3(omega)
  "u1  "/1 -> Unit Delay5/1
  MATLAB Function2/2(y2_k) -> Unit Delay4/1, Gain2/1
  Unit Delay4/1 -> MATLAB Function2/5(y2_k_1)
  Unit Delay5/1 -> MATLAB Function2/2(u1_k_1)
  MATLAB Function2/1(y1_k) -> Unit Delay3/1
  Unit Delay3/1 -> MATLAB Function2/4(y1_k_1)

== system UPI_CC_3ph_4w_seq_23b/Seq_Decom 1/alpha-beta_fasea_LPF1 ==
  u1 : Inport
  omega : Inport  Port=2
  Gain2 : Gain  Gain=2
  MATLAB Function2 : MATLAB Function  TreatAsAtomicUnit=on
  Mux1 : Mux  Inputs=2
  Unit Delay3 : UnitDelay  SampleTime=50e-6  HasFrameUpgradeWarning=on
  Unit Delay4 : UnitDelay  SampleTime=50e-6  HasFrameUpgradeWarning=on
  Unit Delay5 : UnitDelay  SampleTime=50e-6  HasFrameUpgradeWarning=on
  "u1  " : InportShadow
  alpha_beta : Outport
  wires:
  Unit Delay3/1 -> MATLAB Function2/4(y1_k_1)
  MATLAB Function2/1(y1_k) -> Unit Delay3/1
  Unit Delay5/1 -> MATLAB Function2/2(u1_k_1)
  Unit Delay4/1 -> MATLAB Function2/5(y2_k_1)
  MATLAB Function2/2(y2_k) -> Gain2/1, Unit Delay4/1
  "u1  "/1 -> Unit Delay5/1
  omega/1 -> MATLAB Function2/3(omega)
  Gain2/1 -> Mux1/2
  u1/1 -> Mux1/1, MATLAB Function2/1(u1)
  Mux1/1 -> alpha_beta/1

== matlab function UPI_CC_3ph_4w_seq_23b/Control PI_VC/MATLAB Function1 ==
  data: theta input size=1; dq output; abc input
function dq  = fcn(theta,abc)
%#codegen

T_p = 2.0/3.0*[[ cos(theta), cos(theta-2.0/3.0*pi), cos(theta+2.0/3.0*pi)];
               [-sin(theta),-sin(theta-2.0/3.0*pi),-sin(theta+2.0/3.0*pi)]];
           
dq=T_p*abc;

== matlab function UPI_CC_3ph_4w_seq_23b/Control PI_VC/MATLAB Function2 ==
  data: theta input size=1; dq output; abc input
function dq  = fcn(theta,abc)
%#codegen

T_p = 2.0/3.0*[[ cos(theta), cos(theta-2.0/3.0*pi), cos(theta+2.0/3.0*pi)];
               [-sin(theta),-sin(theta-2.0/3.0*pi),-sin(theta+2.0/3.0*pi)]];
           
dq=T_p*abc;
